simulink model "aae301hw08fig56v2"  (R2016a)
settings: Solver=FixedStepAuto  StartTime=0.0  StopTime=12.0  FixedStep=0.001  RelTol=1e-3
settings Model: Creator=mayer15  LastModifiedBy=mayer15

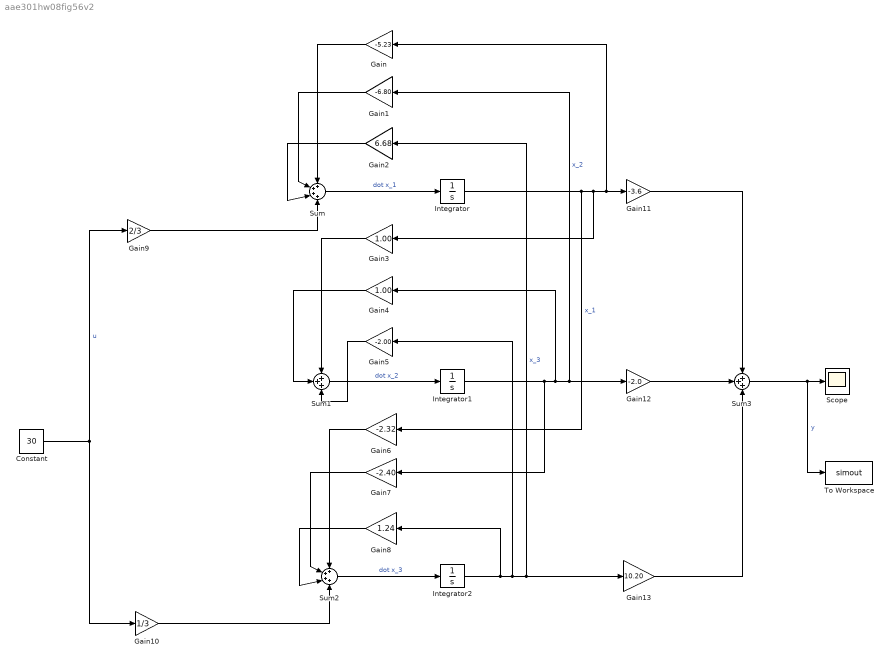
== system aae301hw08fig56v2 ==
  Constant : Constant  Value=30
  Gain : Gain  Gain=-5.23
  Gain1 : Gain  Gain=-6.80
  Gain10 : Gain  Gain=1/3
  Gain11 : Gain  Gain=-3.6
  Gain12 : Gain  Gain=-2.0
  Gain13 : Gain  Gain=10.20
  Gain2 : Gain  Gain=6.68
  Gain3 : Gain  Gain=1.00
  Gain4 : Gain  Gain=1.00
  Gain5 : Gain  Gain=-2.00
  Gain6 : Gain  Gain=-2.32
  Gain7 : Gain  Gain=-2.40
  Gain8 : Gain  Gain=1.24
  Gain9 : Gain  Gain=2/3
  Integrator : Integrator
  Integrator1 : Integrator
  Integrator2 : Integrator
  Scope : Scope
  Sum : Sum  Inputs=++++
  Sum1 : Sum  Inputs=+++
  Sum2 : Sum  Inputs=++++
  Sum3 : Sum  Inputs=+++
  To Workspace : ToWorkspace  VariableName=simout  SampleTime=-1
      settings: Save2DSignal=2-D array (concatenate along first dimension)
  wires:
  Sum1/1 -> Integrator1/1  "dot x_2"
  Sum/1 -> Integrator/1  "dot x_1"
  Sum2/1 -> Integrator2/1  "dot x_3"
  Constant/1 -> Gain9/1, Gain10/1  "u"
  Gain9/1 -> Sum/4
  Gain10/1 -> Sum2/4
  Integrator/1 -> Gain6/1, Gain3/1, Gain/1, Gain11/1  "x_1"
  Integrator1/1 -> Gain7/1, Gain4/1, Gain1/1, Gain12/1  "x_2"
  Integrator2/1 -> Gain8/1, Gain5/1, Gain2/1, Gain13/1  "x_3"
  Sum3/1 -> To Workspace/1, Scope/1  "y"
  Gain11/1 -> Sum3/1
  Gain12/1 -> Sum3/2
  Gain13/1 -> Sum3/3
  Gain/1 -> Sum/1
  Gain1/1 -> Sum/2
  Gain2/1 -> Sum/3
  Gain3/1 -> Sum1/1
  Gain4/1 -> Sum1/2
  Gain5/1 -> Sum1/3
  Gain6/1 -> Sum2/1
  Gain7/1 -> Sum2/2
  Gain8/1 -> Sum2/3
